simulink model "Exemplo2"  (R2021a)
settings: Solver=VariableStepAuto  StartTime=0.0  StopTime=10.0  MaxStep=100  RelTol=1e-3
values from neighbouring files (symbols this model uses):
  g = 10    [script.m]
  k = 10    [script.m]
  l = 1    [script.m]
  m = 10    [script.m]
settings Model: Creator=taffarel55  LastModifiedBy=taffarel55

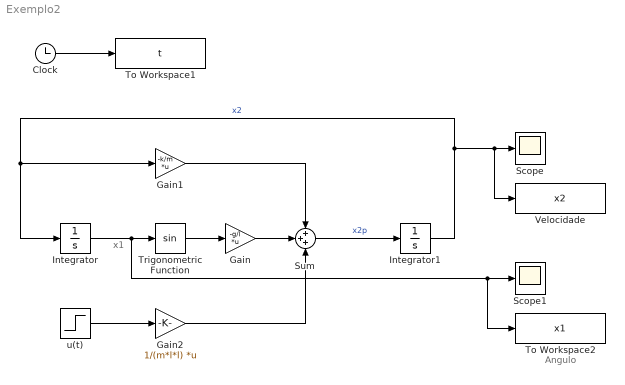
== system Exemplo2 ==
  note: Angulo
  note: x1
  Clock : Clock
  Gain : Gain  Gain=-g/l  Multiplication=Matrix(K*u)
  Gain1 : Gain  Gain=-k/m  Multiplication=Matrix(K*u)
  Gain2 : Gain  Gain=1/(m*l*l)  Multiplication=Matrix(K*u)
  Integrator : Integrator
  Integrator1 : Integrator
  Scope : Scope
  Scope1 : Scope
  Sum : Sum  Inputs=+++
  To Workspace1 : ToWorkspace  VariableName=t  SaveFormat=Timeseries  SampleTime=-1
  To Workspace2 : ToWorkspace  VariableName=x1  SampleTime=-1
  Trigonometric Function : Trigonometry
  Velocidade : ToWorkspace  VariableName=x2  SampleTime=-1
  u(t) : Step  Time=0  SampleTime=0
  wires:
  Clock/1 -> To Workspace1/1
  Integrator/1 -> To Workspace2/1, Scope1/1, Trigonometric Function/1
  Trigonometric Function/1 -> Gain/1
  Gain/1 -> Sum/2
  Gain1/1 -> Sum/1
  u(t)/1 -> Gain2/1
  Gain2/1 -> Sum/3
  Sum/1 -> Integrator1/1  "x2p"
  Integrator1/1 -> Velocidade/1, Scope/1, Integrator/1, Gain1/1  "x2"
